simulink model "delays"  (R2024b)
settings: Solver=VariableStepAuto  StartTime=0.0  StopTime=10.0  RelTol=1e-3
settings Model: Creator=ryandavis  LastModifiedBy=ryandavis

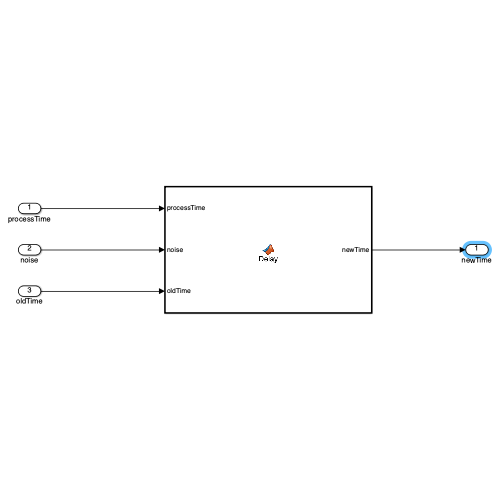
[thumbnail: Simulink's stored preview of the top-level diagram]
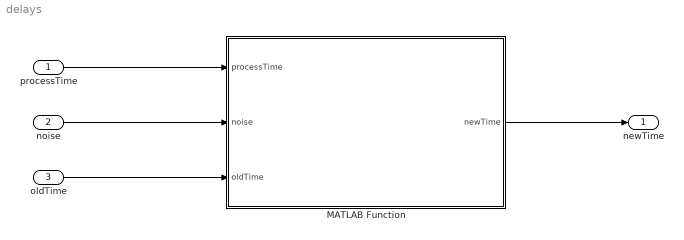
== system delays ==
  processTime : Inport
  noise : Inport  Port=2
  oldTime : Inport  Port=3
  MATLAB Function : MATLAB Function  TreatAsAtomicUnit=on
  newTime : Outport
  wires:
  processTime/1 -> MATLAB Function/1(processTime)
  noise/1 -> MATLAB Function/2(noise)
  oldTime/1 -> MATLAB Function/3(oldTime)
  MATLAB Function/1(newTime) -> newTime/1

== matlab function delays/MATLAB Function ==
  data: processTime input; newTime output; noise input; oldTime input
function newTime= Delay(processTime, noise, oldTime)
if nargain<2
    noise=0;
    oldTime= 0;
elseif nargin<3
    oldTime=0;
end

if oldTime<0
    newTime=-1
else
    newTime= max(oldTime+processTime+noise, 0);
end
